simulink model "sim_emt"  (R2025a)
settings: Solver=ode23s  StartTime=0.0  StopTime=3  RelTol=1e-3
undefined symbols (not defined in the file): bus, gfli_a, inf_src, line_pi, ts
libraries: sps_library x5, sps_lib x1
settings Model: SimulationMode=accelerator  Creator=sern494  LastModifiedBy=paul

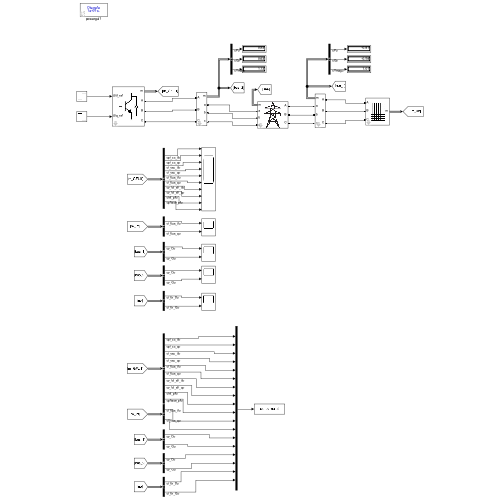
[thumbnail: Simulink's stored preview of the top-level diagram]
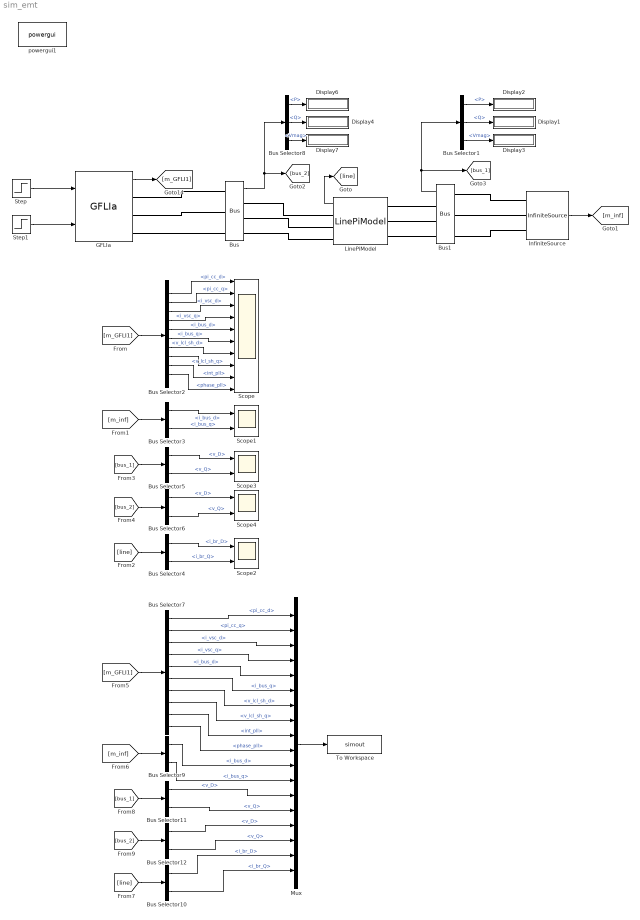
== system sim_emt ==
  Bus : sps_library/Bus  s=bus{1}  sbase=100000000  vbase=230000  fbase=60
  Bus Selector1 : BusSelector  OutputSignals=P,Q,Vmag
  Bus Selector10 : BusSelector  OutputSignals=i_br_D,i_br_Q
  Bus Selector{5..6,11..12} (4 alike) : BusSelector  OutputSignals=v_D,v_Q
  Bus Selector2 : BusSelector  OutputSignals=pi_cc_d,pi_cc_q,i_vsc_d,i_vsc_q,i_bus_d,i_bus_q,v_lcl_sh_d,v_lcl_sh_q,int_pll,phase_pll
  Bus Selector3 : BusSelector  OutputSignals=i_bus_d,i_bus_q
  Bus Selector4 : BusSelector  OutputSignals=i_br_D,i_br_Q
  Bus Selector7 : BusSelector  OutputSignals=pi_cc_d,pi_cc_q,i_vsc_d,i_vsc_q,i_bus_d,i_bus_q,v_lcl_sh_d,v_lcl_sh_q,int_pll,phase_pll
  Bus Selector8 : BusSelector  OutputSignals=P,Q,Vmag
  Bus Selector9 : BusSelector  OutputSignals=i_bus_d,i_bus_q
  Bus1 : sps_library/Bus  s=bus{1}  sbase=100000000  vbase=230000  fbase=60
  Display{1..4,6..7} (6 alike) : Display
      settings: Format=bank
  GFLIa : sps_library/GFLIa  s=gfli_a{1}
  InfiniteSource : sps_library/InfiniteSource  s=inf_src{1}
  LinePiModel : sps_library/LinePiModel  s=line_pi{1}
  Mux : Mux  Inputs=18
  Scope : Scope  NumInputPorts=10
      settings: ActiveDisplayYMinimum=0.29831515666971364  ActiveDisplayYMaximum=0.32536267664692897  DataLoggingVariableName=ScopeData2
  Scope{1..4} (4 alike) : Scope  NumInputPorts=2
      Scope3 settings: ActiveDisplayYMinimum=0.77320547975268017  ActiveDisplayYMaximum=1.021688575630993  DataLoggingVariableName=ScopeData3
      Scope4 settings: DataLoggingVariableName=ScopeData4
  Step : Step  Time=0.3  After=0.1  SampleTime=0
  Step1 : Step  Time=2  After=-0.1  SampleTime=0
  To Workspace : ToWorkspace  VariableName=simout  SaveFormat=Timeseries  SampleTime=10^(-3)
  powergui1 : sps_lib/powergui  Priority=1  SimulationMode=Discrete  SampleTime=ts  frequency=60  Iterations=50  frequencyindice=0  Pbase=100e6  ErrMax=1e-4  UnitsV=kV  UnitsW=MW  buscounter=0  FunctionMessages=off  echomessages=off  EnableUseOfTLC=off  CurrentSourceSwitches=off  DisableSnubberDevices=off  DisableRonSwitches=off  DisableVfSwitches=off  DisplayEquations=off  AutomaticDiscreteSolvers=off  SolverType=Tustin/Backward Euler (TBE)  Interpol=off  ExternalGateDelay=off  methode=off  Ts=100  x0status=blocks  SPID=on  SwTol=0  HookPort=off  NonlinearTolerance=1e-4  nMaxIteration=100  ContinueOnMaxIteration=off  RestoreLinks=warning  ResistiveCurrentMeasurement=off  Frange=[0:2:500]  Ylog=off  Xlog=on  ShowGrid=off  save=off  variable=ZData  structure=0  ZoomFFT=off  StartTime=0.0  cycles=1  DisplayStyle=1  fundamental=60  FreqAxis=off  MaxFrequency=1000  frequencyindicesteady=1  RmsSteady=1  display=off
  wires:
  Bus Selector8/3 -> Display7/1  "<Vmag>"
  Bus Selector8/2 -> Display4/1  "<Q>"
  Bus Selector8/1 -> Display6/1  "<P>"
  Bus Selector1/1 -> Display2/1  "<P>"
  Bus Selector1/2 -> Display1/1  "<Q>"
  Bus Selector1/3 -> Display3/1  "<Vmag>"
  GFLIa/1 -> [m_GFLI1]
  [m_GFLI1] -> Bus Selector2/1
  InfiniteSource/1 -> [m_inf]
  Bus/1 -> [bus_2], Bus Selector8/1
  Bus1/1 -> [bus_1], Bus Selector1/1
  [m_inf] -> Bus Selector3/1
  Bus Selector3/1 -> Scope1/1  "<i_bus_d>"
  Bus Selector3/2 -> Scope1/2  "<i_bus_q>"
  LinePiModel/1 -> [line]
  [line] -> Bus Selector4/1
  Bus Selector4/1 -> Scope2/1  "<i_br_D>"
  Bus Selector4/2 -> Scope2/2  "<i_br_Q>"
  [bus_1] -> Bus Selector5/1
  [bus_2] -> Bus Selector6/1
  Bus Selector5/1 -> Scope3/1  "<v_D>"
  Bus Selector5/2 -> Scope3/2  "<v_Q>"
  Bus Selector6/1 -> Scope4/1  "<v_D>"
  Bus Selector6/2 -> Scope4/2  "<v_Q>"
  [m_inf] -> Bus Selector9/1
  Bus Selector9/1 -> Mux/11  "<i_bus_d>"
  [line] -> Bus Selector10/1
  [m_GFLI1] -> Bus Selector7/1
  Bus Selector9/2 -> Mux/12  "<i_bus_q>"
  [bus_2] -> Bus Selector12/1
  [bus_1] -> Bus Selector11/1
  Mux/1 -> To Workspace/1
  Bus Selector10/1 -> Mux/17  "<i_br_D>"
  Bus Selector10/2 -> Mux/18  "<i_br_Q>"
  Bus Selector11/1 -> Mux/13  "<v_D>"
  Bus Selector11/2 -> Mux/14  "<v_Q>"
  Bus Selector12/1 -> Mux/15  "<v_D>"
  Bus Selector12/2 -> Mux/16  "<v_Q>"
  Bus Selector2/1 -> Scope/1  "<pi_cc_d>"
  Bus Selector2/2 -> Scope/2  "<pi_cc_q>"
  Bus Selector2/3 -> Scope/3  "<i_vsc_d>"
  Bus Selector2/4 -> Scope/4  "<i_vsc_q>"
  Bus Selector2/5 -> Scope/5  "<i_bus_d>"
  Bus Selector2/6 -> Scope/6  "<i_bus_q>"
  Bus Selector2/7 -> Scope/7  "<v_lcl_sh_d>"
  Bus Selector2/8 -> Scope/8  "<v_lcl_sh_q>"
  Bus Selector2/9 -> Scope/9  "<int_pll>"
  Bus Selector2/10 -> Scope/10  "<phase_pll>"
  Bus Selector7/1 -> Mux/1  "<pi_cc_d>"
  Bus Selector7/2 -> Mux/2  "<pi_cc_q>"
  Bus Selector7/3 -> Mux/3  "<i_vsc_d>"
  Bus Selector7/4 -> Mux/4  "<i_vsc_q>"
  Bus Selector7/5 -> Mux/5  "<i_bus_d>"
  Bus Selector7/6 -> Mux/6  "<i_bus_q>"
  Bus Selector7/7 -> Mux/7  "<v_lcl_sh_d>"
  Bus Selector7/8 -> Mux/8  "<v_lcl_sh_q>"
  Bus Selector7/9 -> Mux/9  "<int_pll>"
  Bus Selector7/10 -> Mux/10  "<phase_pll>"
  Step/1 -> GFLIa/1
  Step1/1 -> GFLIa/2
  connections:
  GFLIa/RConn1 -- Bus/LConn1
  GFLIa/RConn2 -- Bus/LConn2
  GFLIa/RConn3 -- Bus/LConn3
  Bus1/LConn1 -- InfiniteSource/LConn1
  Bus1/LConn2 -- InfiniteSource/LConn2
  Bus1/LConn3 -- InfiniteSource/LConn3
  LinePiModel/LConn1 -- Bus1/RConn1
  LinePiModel/LConn2 -- Bus1/RConn2
  LinePiModel/LConn3 -- Bus1/RConn3
  LinePiModel/RConn1 -- Bus/RConn1
  Bus/RConn2 -- LinePiModel/RConn2
  Bus/RConn3 -- LinePiModel/RConn3
